simulink model "Divide"  (R2020a)
settings: Solver=VariableStepAuto  StartTime=0.0  StopTime=10.0  RelTol=1e-3
settings Model: Creator=royde  LastModifiedBy=royde

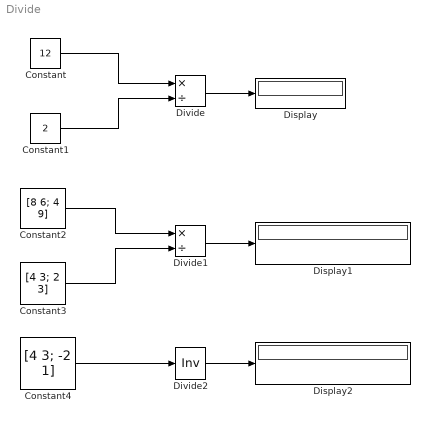
== system Divide ==
  Constant : Constant  Value=12
  Constant1 : Constant  Value=2
  Constant2 : Constant  Value=[8 6; 4 9]
  Constant3 : Constant  Value=[4 3; 2 3]
  Constant4 : Constant  Value=[4 3; -2 1]
  Display : Display
  Display1 : Display
  Display2 : Display
  Divide : Product  Inputs=*/
  Divide1 : Product  Inputs=*/
  Divide2 : Product  Inputs=/  Multiplication=Matrix(*)
  wires:
  Constant/1 -> Divide/1
  Constant1/1 -> Divide/2
  Divide/1 -> Display/1
  Divide1/1 -> Display1/1
  Constant3/1 -> Divide1/2
  Constant2/1 -> Divide1/1
  Constant4/1 -> Divide2/1
  Divide2/1 -> Display2/1
